simulink model "commqpsktxrx"  (R2023b)
settings: Solver=FixedStepDiscrete  StartTime=0.0  StopTime=50  FixedStep=qpsktxrx.FrameTime  RelTol=1e-3
PreLoadFcn:
  | qpsktxrx = commqpsktxrx_init();
InitFcn:
  | qpsktxrx = commqpsktxrx_init();
  | load('n4s1.mat')
StartFcn:
  | load('n4s1.mat')
StopFcn:
  | if (strcmp(get_param([bdroot, '/Model Parameters'],'ShowRecvMsg'),'on'))
  |   if exist('Received','var')
  |      fprintf('%s', Received.signals.values);
  |   end
  | end
libraries: neural x134, dspstat3 x4, simulink x3, dspsigops x3, commdigbbndpm3 x3, commrflib2 x2, commrfcorlib x2, commsequence2 x2, dspsrcs4 x2, commsync2 x2, commfilt2 x2, commchan3 x1
(part 4 of 4)

== system commqpsktxrx/Function Fitting Neural Network/Layer 2/Delays 1 ==
  "p{2}" : Inport  PortDimensions=128
      mask Display: e = 0.06;c1 = [120 230 180]/255;c2 = ([120 230 180]+0)/(256+128);c3 = ([120 230 180]+128)/(256+128);patch([0 1 1 0],[0 0 1 1],c1);patch([0 1 1 1-e 1-e 0+e],[0 0 1 1-e 0+e 0+e],c2);patch([0 0 1 1-e 0+e 0+e],[0 1 1 1-e 1-e 0+e],c3);plot([0 1 1 0 0],[0 0 1 1 0]);
  mux : Mux  Inputs=1
      mask Display: e = 0.06;c1 = [120 150 230]/255;c2 = ([120 150 230]+0)/383;c3 = ([120 150 230]+128)/383;patch([0 1 1 0],[0 0 1 1],c1);patch([0 1 1 1-e 1-e 0+e],[0 0 1 1-e 0+e 0+e],c2);patch([0 0 1 1-e 0+e 0+e],[0 1 1 1-e 1-e 0+e],c3);plot([0 1 1 0 0],[0 0 1 1 0]);disp('Mux')
  "pd{2,1}" : Outport
      mask Display: e = 0.06;c1 = [120 230 180]/255;c2 = ([120 230 180]+0)/(256+128);c3 = ([120 230 180]+128)/(256+128);patch([0 1 1 0],[0 0 1 1],c1);patch([0 1 1 1-e 1-e 0+e],[0 0 1 1-e 0+e 0+e],c2);patch([0 0 1 1-e 0+e 0+e],[0 1 1 1-e 1-e 0+e],c3);plot([0 1 1 0 0],[0 0 1 1 0]);
  wires:
  "p{2}"/1 -> mux/1
  mux/1 -> "pd{2,1}"/1

== system commqpsktxrx/Function Fitting Neural Network/Layer 2/LW{2,1} ==
  "ad{2,1}" : Inport  PortDimensions=128
      mask Display: e = 0.06;c1 = [120 230 180]/255;c2 = ([120 230 180]+0)/(256+128);c3 = ([120 230 180]+128)/(256+128);patch([0 1 1 0],[0 0 1 1],c1);patch([0 1 1 1-e 1-e 0+e],[0 0 1 1-e 0+e 0+e],c2);patch([0 0 1 1-e 0+e 0+e],[0 1 1 1-e 1-e 0+e],c3);plot([0 1 1 0 0],[0 0 1 1 0]);
  "IW{2,1}(1,:)'" : Constant  Value=[-0.08678269051478339213279156183489249087870121002197265625;0.340635837711217248635620080676744692027568817138671875;-0.465263180380636576227715295317466370761394500732421875;-0.9131550023771073387734986681607551872730255126953125;0.94524197252483332931660697795450687408447265625;0.47985714162565817897387887569493614137172698974609375;0.261900590233343610879757079601404257118701934814453125;0.7534990222347233146393818969954736530780792236328125;-0.80736019882414045145679892812040634453296661376953125;0.82163640756908040696515627132612280547618865966796875;0.7368714992051044188059449879801832139492034912109375;0.1561072887199552450265827019393327645957469940185546875;0.444073422703244846676540191765525378286838531494140625;-0.291716419159186723941701302464934997260570526123046875;-0.9377197940791848207453540453570894896984100341796875;-0.389962255790267275923355327904573641717433929443359375;-0.321171281673357789099298997825826518237590789794921875;0.7921137942971883116882736430852673947811126708984375;-0.6164014450186969806821934980689547955989837646484375;-0.364761992917255584156777103999047540128231048583984375;0.1372558127253691029334703443964826874434947967529296875;-0.34139905129450109910749233677051961421966552734375;0.48127058117501075873434501772862859070301055908203125;0.8690896555033902348696983608533628284931182861328125;0.93598971802991837165563993039540946483612060546875;0.9318995711333502018902663621702231466770172119140625;0.38326670891720293621318660370889119803905487060546875;0.1796809873060745965656082034911378286778926849365234375;0.1978454675339807733447372584123513661324977874755859375;0.170206352995841136976906682320986874401569366455078125;-0.01102349793534578535625367834427379420958459377288818359375;-0.516719447107794049856011042720638215541839599609375;-0.1251090024138265255349011795260594226419925689697265625;-0.0029212003527703429839323945316209574230015277862548828125;0.4683787361594575759937697512214072048664093017578125;-0.4369802894019816363879726850427687168121337890625;-0.79299330205270857074850709977908991277217864990234375;0.2225012058753007837541559865712770260870456695556640625;-0.0758165655126610271707932042772881686687469482421875;-0.021638249025532969860297072273169760592281818389892578125;0.5755032126102996858918459111009724438190460205078125;0.8273414033527004551871186777134425938129425048828125;-0.415511199989050117320488197947270236909389495849609375;-0.84410319977900838406270622726879082620143890380859375;0.88107721869636834721717377760796807706356048583984375;0.658593547868766560071662752307020127773284912109375;0.129992024491109858796988874019007198512554168701171875;0.7210963404213865945990846739732660353183746337890625;-0.1808398143561689985769902477841242216527462005615234375;-0.433988785415128919265015383643913082778453826904296875;0.42389226671329272022603618097491562366485595703125;-0.2470524853422368105615447575473808683454990386962890625;0.5575133168413970441434912572731263935565948486328125;-0.305946404386954140530718859736225567758083343505859375;-0.223010039929051939733284370959154330193996429443359375;-0.72491694851056143189538261140114627778530120849609375;0.74301068982151241559819254689500667154788970947265625;-0.242599717969533335004683749502873979508876800537109375;-0.0025082696800795474013912045307961307116784155368804931640625;-0.000620781073481542510807129620076239007175900042057037353515625;0.00022885329768781349931393298557935622739023528993129730224609375;-0.00056896973592614869495720508751901434152387082576751708984375;-0.00038451415643524244382389642993302913964726030826568603515625;0.00054249728227263285980364049265745052252896130084991455078125;0.000595000405852303087921029156603935916791670024394989013671875;0.000622113458333186926212110545719724541413597762584686279296875;-0.000820847325831875894615319300129385737818665802478790283203125;-0.0004060232855676053549155712918405924938269890844821929931640625 ...(+3631 chars)]
      mask Display: e = 0.06;c1 = [120 150 230]/255;c2 = ([120 150 230]+0)/383;c3 = ([120 150 230]+128)/383;patch([0 1 1 0],[0 0 1 1],c1);patch([0 1 1 1-e 1-e 0+e],[0 0 1 1-e 0+e 0+e],c2);patch([0 0 1 1-e 0+e 0+e],[0 1 1 1-e 1-e 0+e],c3);plot([0 1 1 0 0],[0 0 1 1 0]);disp('weights');
  Mux : Mux  Inputs=1
      mask Display: e = 0.06;c1 = [120 150 230]/255;c2 = ([120 150 230]+0)/383;c3 = ([120 150 230]+128)/383;patch([0 1 1 0],[0 0 1 1],c1);patch([0 1 1 1-e 1-e 0+e],[0 0 1 1-e 0+e 0+e],c2);patch([0 0 1 1-e 0+e 0+e],[0 1 1 1-e 1-e 0+e],c3);plot([0 1 1 0 0],[0 0 1 1 0]);disp('Mux');
  dotprod1 : neural/Weight Functions/dotprod
  "lz{2,1}" : Outport
      mask Display: e = 0.06;c1 = [120 230 180]/255;c2 = ([120 230 180]+0)/(256+128);c3 = ([120 230 180]+128)/(256+128);patch([0 1 1 0],[0 0 1 1],c1);patch([0 1 1 1-e 1-e 0+e],[0 0 1 1-e 0+e 0+e],c2);patch([0 0 1 1-e 0+e 0+e],[0 1 1 1-e 1-e 0+e],c3);plot([0 1 1 0 0],[0 0 1 1 0]);
  wires:
  "IW{2,1}(1,:)'"/1 -> dotprod1/1
  "ad{2,1}"/1 -> dotprod1/2
  dotprod1/1 -> Mux/1
  Mux/1 -> "lz{2,1}"/1

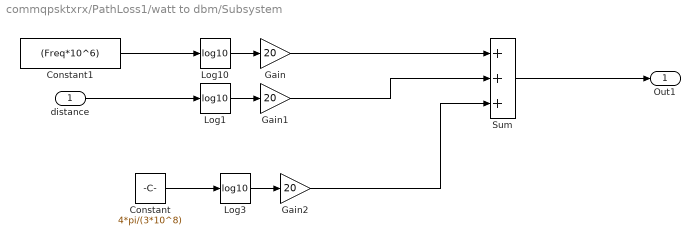
== system commqpsktxrx/PathLoss1/watt to dbm/Subsystem ==
  distance : Inport
  Constant : Constant  Value=4*pi/(3*10^8)
  Constant1 : Constant  Value=(Freq*10^6)
  Gain : Gain  Gain=20
  Gain1 : Gain  Gain=20
  Gain2 : Gain  Gain=20
  Log1 : Math  Operator=log10
  Log10 : Math  Operator=log10
  Log3 : Math  Operator=log10
  Sum : Sum  Inputs=+++
  Out1 : Outport
  wires:
  Constant/1 -> Log3/1
  Log3/1 -> Gain2/1
  Gain2/1 -> Sum/3
  Gain1/1 -> Sum/2
  Gain/1 -> Sum/1
  Log1/1 -> Gain1/1
  Log10/1 -> Gain/1
  distance/1 -> Log1/1
  Sum/1 -> Out1/1
  Constant1/1 -> Log10/1

== system commqpsktxrx/PathLoss1/watt to dbm/Subsystem1 ==
  t : Inport
  Abs : Abs  SaturateOnIntegerOverflow=off
  Constant : Constant  Value=max_pos
  Constant1 : Constant  Value=accel_time
  Constant2 : Constant  Value=decel_time
  Constant3 : Constant  Value=qpsktxrx.TotalFrame * qpsktxrx.FrameTime
  MATLAB Function1 : MATLAB Function  TreatAsAtomicUnit=on
  Out1 : Outport
  wires:
  Abs/1 -> Out1/1
  MATLAB Function1/1(pos) -> Abs/1
  Constant2/1 -> MATLAB Function1/4(decel_time)
  Constant1/1 -> MATLAB Function1/3(accel_time)
  Constant/1 -> MATLAB Function1/2(max_pos)
  Constant3/1 -> MATLAB Function1/5(total_time)
  t/1 -> MATLAB Function1/1(t)

== system commqpsktxrx/Receiver/Data Decoding/Barker Code Symbol Generation  ==
  note: Regenerate a QPSK-modulated unipolar Barker code sequence
      | to be compared with the received data
  Constant Barker Code : Constant  Value=(qpsktxrx.BarkerCode)' > 0  VectorParams1D=off  OutDataTypeStr=double
  QPSK Modulator Baseband : commdigbbndpm3/QPSK Modulator Baseband  InType=Bit  Enc=Gray  Ph=pi/4  outDtype=double  outWordLen=16  outUDDataType=sfix(16)  outFracLenMode=Best precision  outFracLen=15  outDataTypeStr=double  outLastDataTypeStr=double
  Repeat : dspsigops/Repeat  FactorSource=Dialog parameter  N=2  Nmax=16  InputProcessing=Columns as channels (frame based)  RateOptions=Enforce single-rate processing  ic=0  mode=Unused parameter value
  Out : Outport  VectorParamsAs1DForOutWhenUnconnected=off
  wires:
  Constant Barker Code/1 -> Repeat/1
  Repeat/1 -> QPSK Modulator Baseband/1
  QPSK Modulator Baseband/1 -> Out/1

== system commqpsktxrx/Receiver/Data Decoding/Descrambling ==
  In : Inport
  Descrambler : commsequence2/Descrambler  M=2  poly=[1 1 1 0 1]  iniStaSource=Dialog Parameter  ini_sta=[0 0 0 0]  resetViaPort=off
  Selector : Selector  IndexOptions=Index vector (dialog)  Indices=[qpsktxrx.HeaderLength+(1 : qpsktxrx.PayloadLength)]  OutputSizes=1
  Out : Outport  VectorParamsAs1DForOutWhenUnconnected=off
  wires:
  In/1 -> Selector/1
  Selector/1 -> Descrambler/1
  Descrambler/1 -> Out/1

== system commqpsktxrx/Receiver/Data Decoding/Phase Ambiguity Correction & Demodulation ==
  note: Phase Ambiguity Resolution
      | and Demodulation
  Phase : Inport
  Data : Inport  Port=2
  Complex Phase Shift : commutil2/Complex Phase Shift
  Gain : Gain  Gain=-1  OutDataTypeStr=Inherit: Same as input
  QPSK Demodulator Baseband : commdigbbndpm3/QPSK Demodulator Baseband  OutType=Bit  DecType=Hard decision  VarSource=Dialog  Variance=1  Dec=Gray  Ph=pi/4  outDtype1=Inherit via internal rule  outDtype2=Inherit via internal rule  derotateFactorWordLen=16  derotateFactorDataTypeStr=Inherit: Same word length as input  derotateFactorLastDataTypeStr=Inherit: Same word length as input
  Out : Outport  VectorParamsAs1DForOutWhenUnconnected=off
  wires:
  Phase/1 -> Gain/1
  Data/1 -> Complex Phase Shift/1
  Complex Phase Shift/1 -> QPSK Demodulator Baseband/1
  QPSK Demodulator Baseband/1 -> Out/1
  Gain/1 -> Complex Phase Shift/2

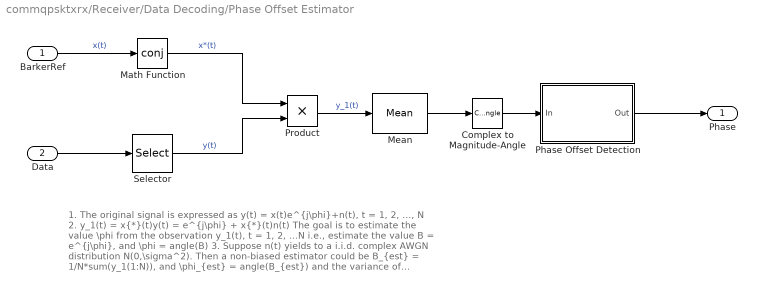
== system commqpsktxrx/Receiver/Data Decoding/Phase Offset Estimator ==
  note: 1. The original signal is expressed as y(t) = x(t)e^{j\phi}+n(t), t = 1, 2, ..., N
      | 2. y_1(t) = x{*}(t)y(t) = e^{j\phi} + x{*}(t)n(t)
      | The goal is to estimate the value \phi from the observation y_1(t), t = 1, 2, ...N
      | i.e., estimate the value B = e^{j\phi}, and \phi = angle(B)
      | 3. Suppose n(t) yields to a i.i.d. complex AWGN distribution N(0,\sigma^2).
      | Then a non-biased estimator could be
      | B_{est} = 1/N*sum(y_1(1:N)), and \phi_{est} = angle(B_{est})
      | and the variance of B_{est} is \sigma^2/N
  BarkerRef : Inport
  Data : Inport  Port=2
  Complex to Magnitude-Angle : ComplexToMagnitudeAngle  Output=Angle
  Math Function : Math  Operator=conj  SignedPower=on
  Mean : dspstat3/Mean  run=off  InputProcessing=Columns as channels (frame based)  reset_popup=None  directionMode=Each column  dimension=1  roiEnable=off  roiType=Rectangles  roiPortion=Entire ROI  roiOutput=Individual statistics for each ROI  roiFlag=off  roundingMode=Floor  overflowMode=off  outputDataTypeStr=Inherit: Same as accumulator  outputMin=[]  outputMax=[]  outputLastDataTypeStr=Inherit: Same as accumulator
  Phase Offset Detection : MATLAB Function  TreatAsAtomicUnit=on
  Product : Product  RndMeth=Zero
  Selector : Selector  IndexOptions=Index vector (dialog)  Indices=[1:qpsktxrx.BarkerLength]  OutputSizes=1
  Phase : Outport  VectorParamsAs1DForOutWhenUnconnected=off
  wires:
  Data/1 -> Selector/1
  BarkerRef/1 -> Math Function/1  "x(t)"
  Selector/1 -> Product/2  "y(t)"
  Math Function/1 -> Product/1  "x*(t)"
  Product/1 -> Mean/1  "y_1(t)"
  Mean/1 -> Complex to Magnitude-Angle/1
  Complex to Magnitude-Angle/1 -> Phase Offset Detection/1(In)
  Phase Offset Detection/1(Out) -> Phase/1

== system commqpsktxrx/Transmitter/Bit Generation/Barker Code SS ==
  Constant Barker Code : Constant  Value=(qpsktxrx.BarkerCode)' > 0; % Bipolar to Unipolar  VectorParams1D=off  OutDataTypeStr=double
  Out : Outport  VectorParamsAs1DForOutWhenUnconnected=off
  wires:
  Constant Barker Code/1 -> Out/1

== matlab function commqpsktxrx/Receiver/Data Decoding/Phase Offset Estimator/Phase Offset Detection ==
  data: In input; Out output
function Out = phasedecision(In)
% Map the estimated phase to one of -pi, -pi/2, 0, pi/2,  
%#codegen
Out = round(In.*2./pi)./2.*pi;
% The above processing is equivalent to the following processing using
% if/else statements
%
% if In<pi/4 && In>-pi/4
%     Out = 0;
% elseif In>=pi/4 && In<pi*3/4
%     Out = pi/2;
% elseif In>=pi*3/4 || In<=-pi*3/4
%     Out = -pi;
% else
%     Out = -pi/2;
% end

== matlab function commqpsktxrx/PathLoss1/watt to dbm/MATLAB Function ==
  data: u input; y output
function y = fcn(u)

y = (10^((-u)/20));

== matlab function commqpsktxrx/Subsystem6/MATLAB Function ==
  data: u input; y output
function y = fcn(u)

y = (10^((u)/20));

== matlab function commqpsktxrx/Subsystem1/MATLAB Function ==
  data: u input; y output
function y = fcn(u)

y = (10^((u)/20));

== matlab function commqpsktxrx/PathLoss1/watt to dbm/Subsystem1/MATLAB Function1 ==
  data: t input; pos output; max_pos input; accel_time input; decel_time input; total_time input
function pos = exponentialPosition(t, max_pos, accel_time, decel_time, total_time)
    % Exponential acceleration and deceleration in position
    % t - current time
    % max_pos - maximum position
    % accel_time - duration of acceleration phase
    % decel_time - duration of deceleration phase
    % total_time - total simulation time
    
    % Define constants for exponential growth
    
    k_accel = 5 / accel_time; % Constant to control exponential growth in acceleration
    k_decel = 5 / decel_time; % Constant to control exponential decay in deceleration
    
    if t < accel_time
        % Acceleration phase (exponential increase)
        pos = 1+max_pos * (1 - exp(-k_accel * t));
    elseif t < (total_time - decel_time)
        % Constant position phase
        pos = 1+ max_pos;
    else
        % Deceleration phase (exponential decrease)
        pos = 1+max_pos * exp(-k_decel * (t - (total_time - decel_time)));
    end
end
